simulink model "ChristophBessler"  (R2017a)
settings: Solver=VariableStepAuto  StartTime=0.0  StopTime=3  RelTol=1e-3
libraries: m3dof_library x12, dspindex x6
settings Model: Creator=Chris  LastModifiedBy=Chris

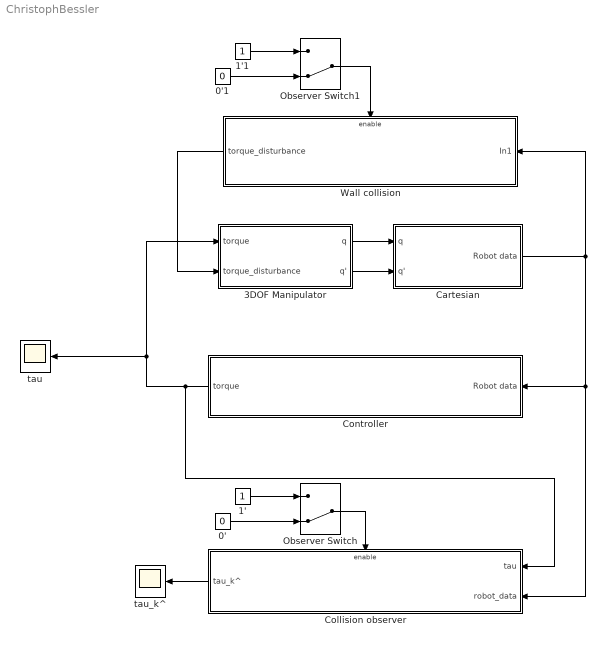
== system ChristophBessler ==
  0' : Constant  Value=0
  0'1 : Constant  Value=0
  1' : Constant
  1'1 : Constant
  3DOF Manipulator : Subsystem
  Cartesian : Subsystem
  Collision observer : Subsystem
  Controller : Subsystem
  Observer Switch : ManualSwitch  CurrentSetting=0
  Observer Switch1 : ManualSwitch  CurrentSetting=0
  Wall collision : Subsystem
  tau : Scope
  tau_k^ : Scope
  wires:
  3DOF Manipulator/1(q) -> Cartesian/1(q)
  3DOF Manipulator/2(q') -> Cartesian/2(q')
  Controller/1(torque) -> Collision observer/1(tau), tau/1, 3DOF Manipulator/1(torque)
  Collision observer/1(tau_k^) -> tau_k^/1
  Cartesian/1(Robot data) -> Wall collision/1(In1), Collision observer/2(robot_data), Controller/1(Robot data)
  Wall collision/1(torque_disturbance) -> 3DOF Manipulator/2(torque_disturbance)
  0'/1 -> Observer Switch/2
  1'/1 -> Observer Switch/1
  Observer Switch/1 -> Collision observer/Enable
  0'1/1 -> Observer Switch1/2
  Observer Switch1/1 -> Wall collision/Enable
  1'1/1 -> Observer Switch1/1

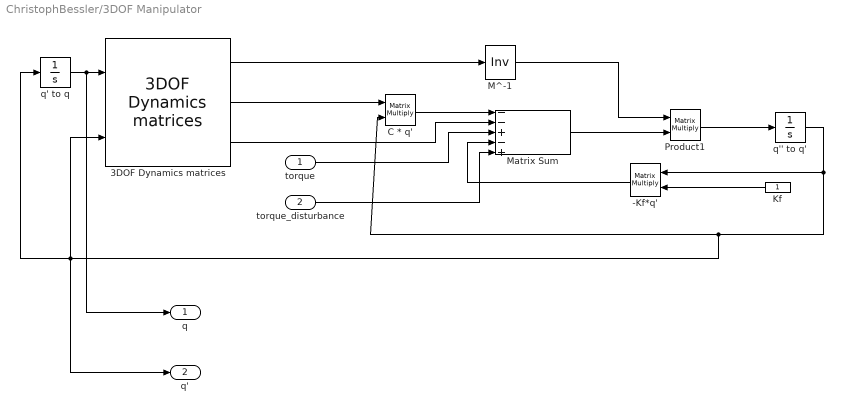
== system ChristophBessler/3DOF Manipulator ==
  torque : Inport
  torque_disturbance : Inport  Port=2
  -Kf*q' : Product  Multiplication=Matrix(*)
  3DOF Dynamics matrices : m3dof_library/3DOF Dynamics matrices  m1=m1  mX1=mx1  ZZ1=I1  m2=m2  mX2=mx2  ZZ2=I2  m3=m3  mX3=mx3  ZZ3=I3  a1=l1  a2=l2  a3=l3  eg=eg
  C * q' : Product  Multiplication=Matrix(*)
  Kf : Constant
  M^-1 : Product  Inputs=/  Multiplication=Matrix(*)
  Matrix Sum : Sum  Inputs=--+-+
  Product1 : Product  Multiplication=Matrix(*)
  q' to q : Integrator  InitialCondition=[3.66519; -0.523599; 0.349066]
  q'' to q' : Integrator
  q : Outport
  q' : Outport  Port=2
  wires:
  q' to q/1 -> q/1, 3DOF Dynamics matrices/1
  M^-1/1 -> Product1/1
  q'' to q'/1 -> -Kf*q'/1, C * q'/2, q'/1, q' to q/1, 3DOF Dynamics matrices/2
  3DOF Dynamics matrices/2 -> C * q'/1
  3DOF Dynamics matrices/1 -> M^-1/1
  Matrix Sum/1 -> Product1/2
  C * q'/1 -> Matrix Sum/1
  Product1/1 -> q'' to q'/1
  3DOF Dynamics matrices/3 -> Matrix Sum/2
  torque/1 -> Matrix Sum/3
  Kf/1 -> -Kf*q'/2
  -Kf*q'/1 -> Matrix Sum/4
  torque_disturbance/1 -> Matrix Sum/5

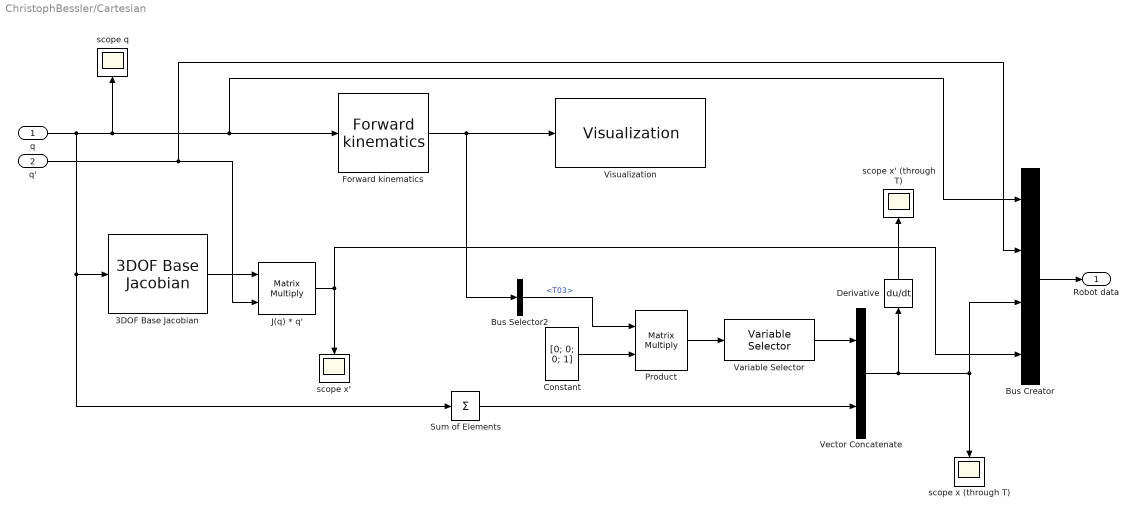
== system ChristophBessler/Cartesian ==
  q : Inport
  q' : Inport  Port=2
  3DOF Base Jacobian : m3dof_library/3DOF Base Jacobian  a1=l1  a2=l2  a3=l3
  Bus Creator : BusCreator  Inputs=4
  Bus Selector2 : BusSelector  OutputSignals=T03
  Constant : Constant  Value=[0; 0; 0; 1]  VectorParams1D=off
  Derivative : Derivative
  Forward kinematics : m3dof_library/Forward kinematics  a1=l1  a2=l2  a3=l3  alpha=0
  J(q) * q' : Product  Multiplication=Matrix(*)
  Product : Product  Multiplication=Matrix(*)
  Sum of Elements : Sum  Inputs=+
  Variable Selector : dspindex/Variable Selector  NumInputs=1  rowsOrCols=Rows  IdxMode=Fixed  Elements=[1 2]  ZerOneIdxMode=One-based  errmode=Clip Index  FillMode=off  FillValues=0
  Vector Concatenate : Concatenate
  Visualization : m3dof_library/Visualization  Ts0=1/16  al=1  a1=l1  a2=l2  a3=l3  alpha=0  eg=eg  tl=50
  scope q : Scope
  scope x (through T) : Scope
  scope x' : Scope
  scope x' (through T) : Scope
  Robot data : Outport
  wires:
  J(q) * q'/1 -> Bus Creator/4, scope x'/1
  3DOF Base Jacobian/1 -> J(q) * q'/1
  Forward kinematics/1 -> Bus Selector2/1, Visualization/1
  Constant/1 -> Product/2
  Variable Selector/1 -> Vector Concatenate/1
  Bus Selector2/1 -> Product/1  "<T03>"
  q/1 -> Sum of Elements/1, 3DOF Base Jacobian/1, Bus Creator/1, Forward kinematics/1, scope q/1
  q'/1 -> Bus Creator/2, J(q) * q'/2
  Vector Concatenate/1 -> Derivative/1, Bus Creator/3, scope x (through T)/1
  Derivative/1 -> scope x' (through T)/1
  Product/1 -> Variable Selector/1
  Bus Creator/1 -> Robot data/1
  Sum of Elements/1 -> Vector Concatenate/2

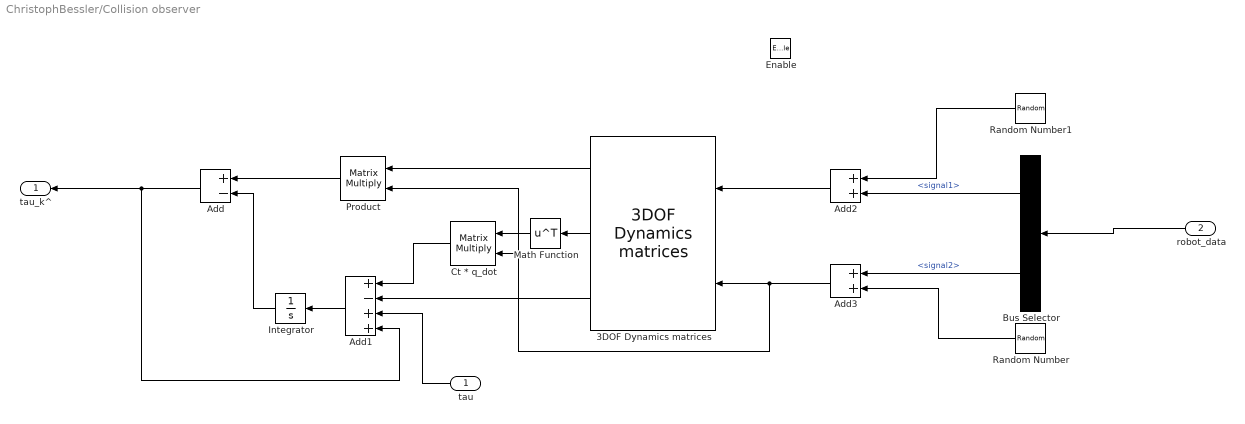
== system ChristophBessler/Collision observer ==
  tau : Inport
  robot_data : Inport  Port=2
  Enable : EnablePort
  3DOF Dynamics matrices : m3dof_library/3DOF Dynamics matrices  m1=m1  mX1=mx1  ZZ1=I1  m2=m2  mX2=mx2  ZZ2=I2  m3=m3  mX3=mx3  ZZ3=I3  a1=l1  a2=l2  a3=l3  eg=eg
  Add : Sum  Inputs=+-
  Add1 : Sum  Inputs=+-++
  Add2 : Sum
  Add3 : Sum
  Bus Selector : BusSelector  OutputSignals=signal1,signal2
  Ct * q_dot : Product  Multiplication=Matrix(*)
  Integrator : Integrator
  Math Function : Math  Operator=transpose  SaturateOnIntegerOverflow=on
  Product : Product  Multiplication=Matrix(*)
  Random Number : RandomNumber  Mean=1  Variance=0.001  SampleTime=0.1
  Random Number1 : RandomNumber  Variance=0.001  SampleTime=0.1
  tau_k^ : Outport
  wires:
  Add2/1 -> 3DOF Dynamics matrices/1
  Add3/1 -> Ct * q_dot/2, Product/2, 3DOF Dynamics matrices/2
  robot_data/1 -> Bus Selector/1
  3DOF Dynamics matrices/1 -> Product/1
  Product/1 -> Add/1
  3DOF Dynamics matrices/3 -> Add1/2
  tau/1 -> Add1/3
  Add1/1 -> Integrator/1
  Integrator/1 -> Add/2
  Bus Selector/1 -> Add2/2  "<signal1>"
  Bus Selector/2 -> Add3/1  "<signal2>"
  Random Number/1 -> Add3/2
  Random Number1/1 -> Add2/1
  3DOF Dynamics matrices/2 -> Math Function/1
  Math Function/1 -> Ct * q_dot/1
  Ct * q_dot/1 -> Add1/1
  Add/1 -> Add1/4, tau_k^/1

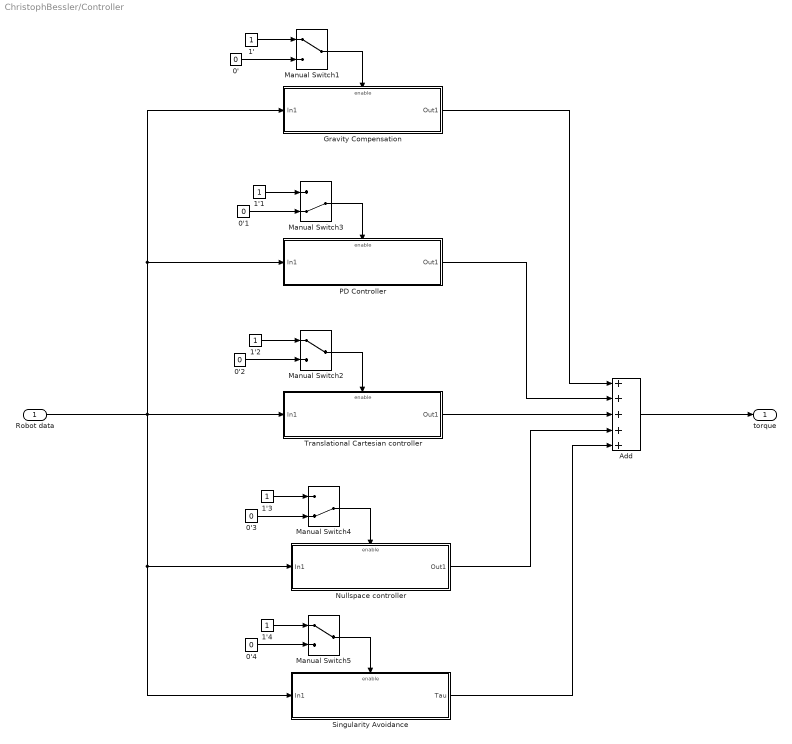
== system ChristophBessler/Controller ==
  Robot data : Inport
  0'{,1..4} (5 alike) : Constant  Value=0
  1'{,1..4} (5 alike) : Constant
  Add : Sum  Inputs=+++++
  Gravity Compensation : Subsystem
  Manual Switch1 : ManualSwitch
  Manual Switch2 : ManualSwitch
  Manual Switch3 : ManualSwitch  CurrentSetting=0
  Manual Switch4 : ManualSwitch  CurrentSetting=0
  Manual Switch5 : ManualSwitch
  Nullspace controller : Subsystem
  PD Controller : Subsystem
  Singularity Avoidance : Subsystem
  Translational Cartesian controller : Subsystem
  torque : Outport
  wires:
  Manual Switch1/1 -> Gravity Compensation/Enable
  Manual Switch3/1 -> PD Controller/Enable
  0'/1 -> Manual Switch1/2
  1'/1 -> Manual Switch1/1
  Add/1 -> torque/1
  1'1/1 -> Manual Switch3/1
  0'1/1 -> Manual Switch3/2
  Gravity Compensation/1(Out1) -> Add/1
  PD Controller/1(Out1) -> Add/2
  1'2/1 -> Manual Switch2/1
  0'2/1 -> Manual Switch2/2
  Manual Switch2/1 -> Translational Cartesian controller/Enable
  Translational Cartesian controller/1(Out1) -> Add/3
  Nullspace controller/1(Out1) -> Add/4
  0'3/1 -> Manual Switch4/2
  1'3/1 -> Manual Switch4/1
  1'4/1 -> Manual Switch5/1
  0'4/1 -> Manual Switch5/2
  Manual Switch4/1 -> Nullspace controller/Enable
  Manual Switch5/1 -> Singularity Avoidance/Enable
  Singularity Avoidance/1(Tau) -> Add/5
  Robot data/1 -> PD Controller/1(In1), Gravity Compensation/1(In1), Singularity Avoidance/1(In1), Nullspace controller/1(In1), Translational Cartesian controller/1(In1)

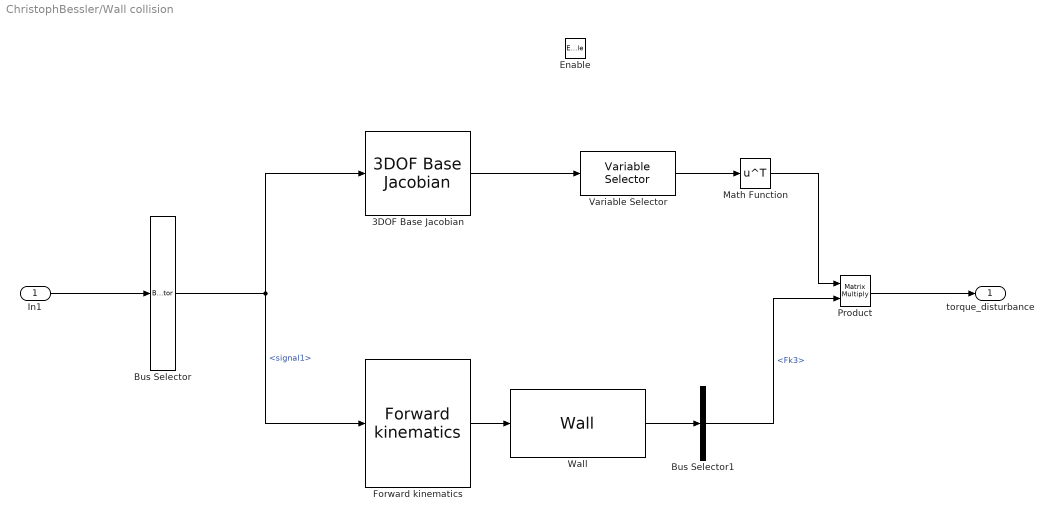
== system ChristophBessler/Wall collision ==
  In1 : Inport
  Enable : EnablePort
  3DOF Base Jacobian : m3dof_library/3DOF Base Jacobian  a1=l1  a2=l2  a3=l3
  Bus Selector : BusSelector  OutputSignals=signal1
  Bus Selector1 : BusSelector  OutputSignals=Fk3
  Forward kinematics : m3dof_library/Forward kinematics  a1=l1  a2=l2  a3=l3  alpha=0
  Math Function : Math  Operator=transpose  SaturateOnIntegerOverflow=on
  Product : Product  Multiplication=Matrix(*)
  Variable Selector : dspindex/Variable Selector  NumInputs=1  rowsOrCols=Rows  IdxMode=Fixed  Elements=[1 2]  ZerOneIdxMode=One-based  errmode=Clip Index  FillMode=on  FillValues=0
  Wall : m3dof_library/Wall  x0=[0 0]  w=[0 -1]
  torque_disturbance : Outport
  wires:
  In1/1 -> Bus Selector/1
  Bus Selector/1 -> Forward kinematics/1, 3DOF Base Jacobian/1  "<signal1>"
  Forward kinematics/1 -> Wall/1
  3DOF Base Jacobian/1 -> Variable Selector/1
  Variable Selector/1 -> Math Function/1
  Product/1 -> torque_disturbance/1
  Math Function/1 -> Product/1
  Wall/1 -> Bus Selector1/1
  Bus Selector1/1 -> Product/2  "<Fk3>"

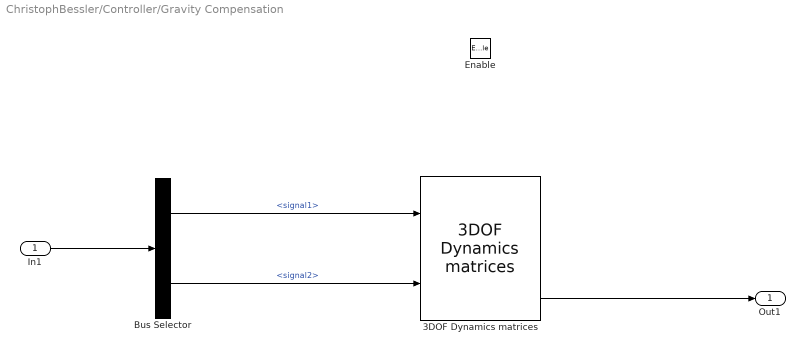
== system ChristophBessler/Controller/Gravity Compensation ==
  In1 : Inport
  Enable : EnablePort
  3DOF Dynamics matrices : m3dof_library/3DOF Dynamics matrices  m1=m1  mX1=mx1  ZZ1=I1  m2=m2  mX2=mx2  ZZ2=I2  m3=m3  mX3=mx3  ZZ3=I3  a1=l1  a2=l2  a3=l3  eg=eg
  Bus Selector : BusSelector  OutputSignals=signal1,signal2
  Out1 : Outport
  wires:
  In1/1 -> Bus Selector/1
  Bus Selector/2 -> 3DOF Dynamics matrices/2  "<signal2>"
  Bus Selector/1 -> 3DOF Dynamics matrices/1  "<signal1>"
  3DOF Dynamics matrices/3 -> Out1/1

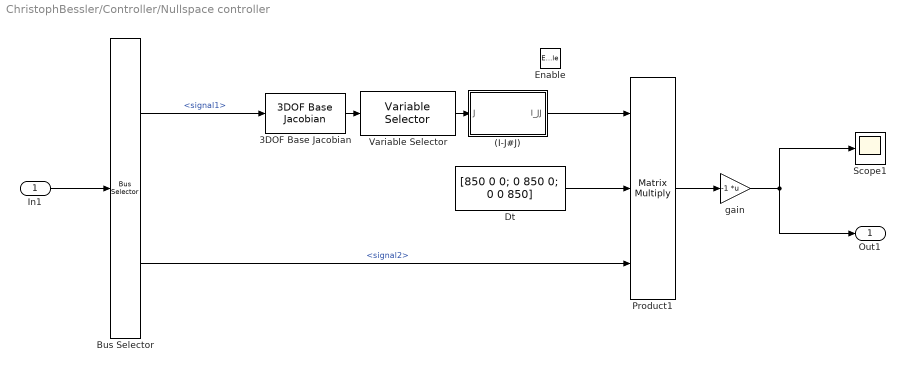
== system ChristophBessler/Controller/Nullspace controller ==
  In1 : Inport
  Enable : EnablePort
  (I-J#J) : MATLAB Function  TreatAsAtomicUnit=on
  3DOF Base Jacobian : m3dof_library/3DOF Base Jacobian  a1=l1  a2=l2  a3=l3
  Bus Selector : BusSelector  OutputSignals=signal1,signal2
  Dt : Constant  Value=[850 0 0; 0 850 0; 0 0 850]
  Product1 : Product  Inputs=3  Multiplication=Matrix(*)
  Scope1 : Scope
  Variable Selector : dspindex/Variable Selector  NumInputs=1  rowsOrCols=Rows  IdxMode=Fixed  Elements=[1 2]  ZerOneIdxMode=One-based  errmode=Clip Index  FillMode=on  FillValues=0
  "gain " : Gain  Gain=-1  Multiplication=Matrix(K*u)
  Out1 : Outport
  wires:
  In1/1 -> Bus Selector/1
  Product1/1 -> "gain "/1
  (I-J#J)/1(I_JJ) -> Product1/1
  "gain "/1 -> Scope1/1, Out1/1
  Bus Selector/1 -> 3DOF Base Jacobian/1  "<signal1>"
  Bus Selector/2 -> Product1/3  "<signal2>"
  Dt/1 -> Product1/2
  3DOF Base Jacobian/1 -> Variable Selector/1
  Variable Selector/1 -> (I-J#J)/1(J)

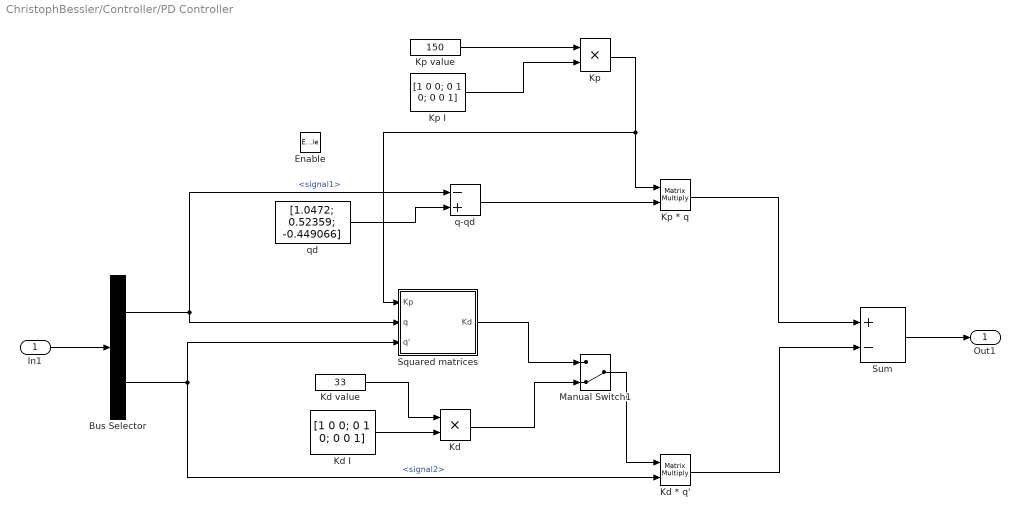
== system ChristophBessler/Controller/PD Controller ==
  In1 : Inport
  Enable : EnablePort
  Bus Selector : BusSelector  OutputSignals=signal1,signal2
  Kd : Product
  Kd * q' : Product  Multiplication=Matrix(*)
  Kd I : Constant  Value=[1 0 0; 0 1 0; 0 0 1]  VectorParams1D=off
  Kd value : Constant  Value=33
  Kp : Product
  Kp * q : Product  Multiplication=Matrix(*)
  Kp I : Constant  Value=[1 0 0; 0 1 0; 0 0 1]  VectorParams1D=off
  Kp value : Constant  Value=150
  Manual Switch1 : ManualSwitch  CurrentSetting=0
  Squared matrices : Subsystem
  Sum : Sum  Inputs=+-
  q-qd : Sum  Inputs=-+
  qd : Constant  Value=[1.0472; 0.52359; -0.449066]  VectorParams1D=off
  Out1 : Outport
  wires:
  In1/1 -> Bus Selector/1
  Bus Selector/1 -> Squared matrices/2(q), q-qd/1  "<signal1>"
  Bus Selector/2 -> Squared matrices/3(q'), Kd * q'/2  "<signal2>"
  Kp * q/1 -> Sum/1
  qd/1 -> q-qd/2
  q-qd/1 -> Kp * q/2
  Kd * q'/1 -> Sum/2
  Kp value/1 -> Kp/1
  Kd I/1 -> Kd/2
  Kd value/1 -> Kd/1
  Kp/1 -> Squared matrices/1(Kp), Kp * q/1
  Kp I/1 -> Kp/2
  Sum/1 -> Out1/1
  Kd/1 -> Manual Switch1/2
  Manual Switch1/1 -> Kd * q'/1
  Squared matrices/1(Kd) -> Manual Switch1/1

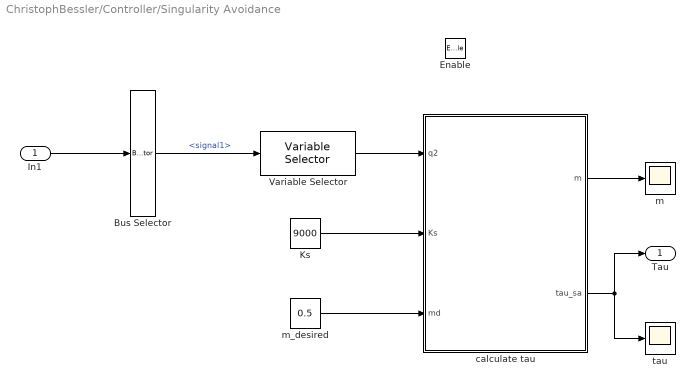
== system ChristophBessler/Controller/Singularity Avoidance ==
  In1 : Inport
  Enable : EnablePort
  Bus Selector : BusSelector  OutputSignals=signal1
  Ks : Constant  Value=9000
  Variable Selector : dspindex/Variable Selector  NumInputs=1  rowsOrCols=Rows  IdxMode=Fixed  Elements=[2]  ZerOneIdxMode=One-based  errmode=Clip Index  FillMode=on  FillValues=0
  calculate tau : MATLAB Function  TreatAsAtomicUnit=on
  m : Scope
  m_desired : Constant  Value=0.5
  tau : Scope
  Tau : Outport
  wires:
  In1/1 -> Bus Selector/1
  Ks/1 -> calculate tau/2(Ks)
  Variable Selector/1 -> calculate tau/1(q2)
  m_desired/1 -> calculate tau/3(md)
  calculate tau/2(tau_sa) -> tau/1, Tau/1
  Bus Selector/1 -> Variable Selector/1  "<signal1>"
  calculate tau/1(m) -> m/1

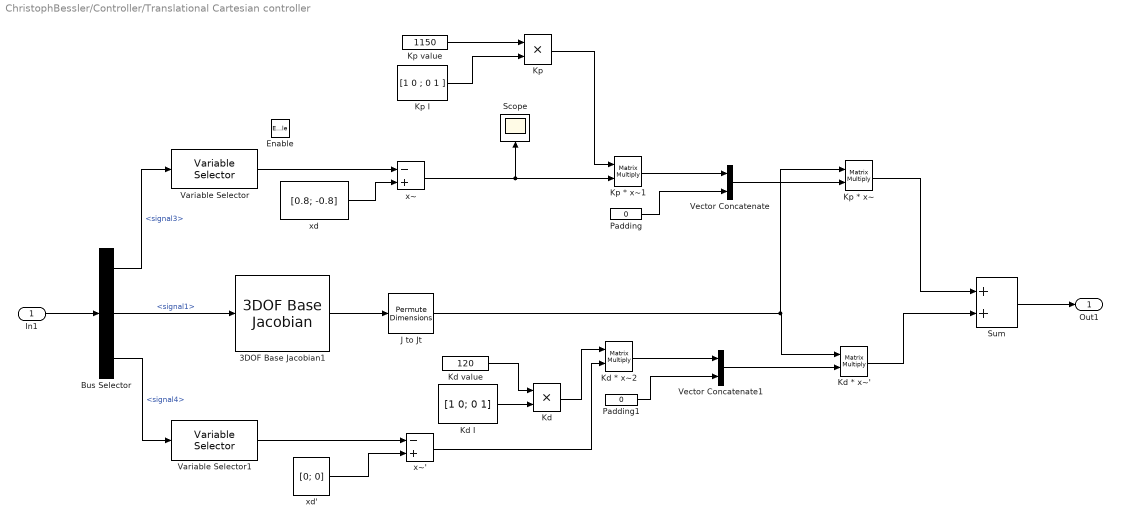
== system ChristophBessler/Controller/Translational Cartesian controller ==
  In1 : Inport
  Enable : EnablePort
  3DOF Base Jacobian1 : m3dof_library/3DOF Base Jacobian  a1=l1  a2=l2  a3=l3
  Bus Selector : BusSelector  OutputSignals=signal3,signal1,signal4
  J to Jt : PermuteDimensions
  Kd : Product
  Kd * x~' : Product  Multiplication=Matrix(*)
  Kd * x~2 : Product  Multiplication=Matrix(*)
  Kd I : Constant  Value=[1 0; 0 1]  VectorParams1D=off
  Kd value : Constant  Value=120
  Kp : Product
  Kp * x~ : Product  Multiplication=Matrix(*)
  Kp * x~1 : Product  Multiplication=Matrix(*)
  Kp I : Constant  Value=[1 0 ; 0 1 ]  VectorParams1D=off
  "Kp value " : Constant  Value=1150
  Padding : Constant  Value=0
  Padding1 : Constant  Value=0
  Scope : Scope
  Sum : Sum
  Variable Selector : dspindex/Variable Selector  NumInputs=1  rowsOrCols=Rows  IdxMode=Fixed  Elements=[1 2]  ZerOneIdxMode=One-based  errmode=Clip Index  FillMode=on  FillValues=0
  Variable Selector1 : dspindex/Variable Selector  NumInputs=1  rowsOrCols=Rows  IdxMode=Fixed  Elements=[1 2]  ZerOneIdxMode=One-based  errmode=Clip Index  FillMode=on  FillValues=0
  Vector Concatenate : Concatenate
  Vector Concatenate1 : Concatenate
  xd : Constant  Value=[0.8; -0.8]  VectorParams1D=off
  xd' : Constant  Value=[0; 0]  VectorParams1D=off
  x~ : Sum  Inputs=-+
  x~' : Sum  Inputs=-+
  Out1 : Outport
  wires:
  In1/1 -> Bus Selector/1
  xd/1 -> x~/2
  Kd * x~'/1 -> Sum/2
  Kd I/1 -> Kd/2
  Kd value/1 -> Kd/1
  Kp I/1 -> Kp/2
  Sum/1 -> Out1/1
  Bus Selector/2 -> 3DOF Base Jacobian1/1  "<signal1>"
  xd'/1 -> x~'/2
  3DOF Base Jacobian1/1 -> J to Jt/1
  Kp * x~/1 -> Sum/1
  J to Jt/1 -> Kp * x~/1, Kd * x~'/1
  Kp/1 -> Kp * x~1/1
  Variable Selector/1 -> x~/1
  Bus Selector/1 -> Variable Selector/1  "<signal3>"
  Variable Selector1/1 -> x~'/1
  Bus Selector/3 -> Variable Selector1/1  "<signal4>"
  Padding/1 -> Vector Concatenate/2
  x~/1 -> Scope/1, Kp * x~1/2
  Kp * x~1/1 -> Vector Concatenate/1
  Vector Concatenate/1 -> Kp * x~/2
  Padding1/1 -> Vector Concatenate1/2
  Vector Concatenate1/1 -> Kd * x~'/2
  Kd * x~2/1 -> Vector Concatenate1/1
  Kd/1 -> Kd * x~2/1
  x~'/1 -> Kd * x~2/2
  "Kp value "/1 -> Kp/1

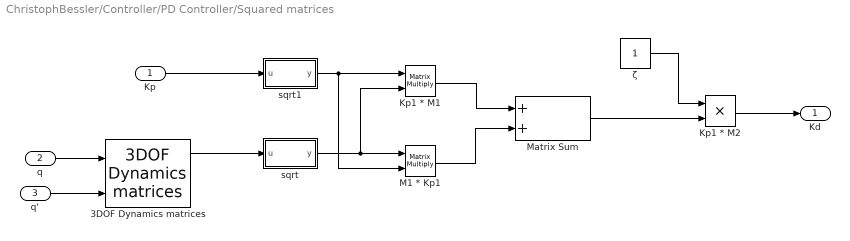
== system ChristophBessler/Controller/PD Controller/Squared matrices ==
  Kp : Inport
  q : Inport  Port=2
  q' : Inport  Port=3
  3DOF Dynamics matrices : m3dof_library/3DOF Dynamics matrices  m1=m1  mX1=mx1  ZZ1=I1  m2=m2  mX2=mx2  ZZ2=I2  m3=m3  mX3=mx3  ZZ3=I3  a1=l1  a2=l2  a3=l3  eg=eg
  Kp1 * M1 : Product  Multiplication=Matrix(*)
  Kp1 * M2 : Product
  M1 * Kp1 : Product  Multiplication=Matrix(*)
  Matrix Sum : Sum
  sqrt : MATLAB Function  TreatAsAtomicUnit=on
  sqrt1 : MATLAB Function  TreatAsAtomicUnit=on
  ζ : Constant
  Kd : Outport
  wires:
  q/1 -> 3DOF Dynamics matrices/1
  Kp/1 -> sqrt1/1(u)
  q'/1 -> 3DOF Dynamics matrices/2
  3DOF Dynamics matrices/1 -> sqrt/1(u)
  sqrt1/1(y) -> M1 * Kp1/2, Kp1 * M1/1
  sqrt/1(y) -> M1 * Kp1/1, Kp1 * M1/2
  Kp1 * M1/1 -> Matrix Sum/1
  M1 * Kp1/1 -> Matrix Sum/2
  Kp1 * M2/1 -> Kd/1
  Matrix Sum/1 -> Kp1 * M2/2
  ζ/1 -> Kp1 * M2/1

== matlab function ChristophBessler/Controller/PD Controller/Squared matrices/sqrt1 ==
  data: u input; y output
function y = fcn(u)

y = real(sqrt(u));

== matlab function ChristophBessler/Controller/PD Controller/Squared matrices/sqrt ==
  data: u input; y output
function y = fcn(u)

y = real(sqrt(u));

== matlab function ChristophBessler/Controller/Nullspace controller/(I-J#J) ==
  data: J input; I_JJ output
function I_JJ = fcn(J)

I_JJ = eye(3)-J'*pinv(J)';

== matlab function ChristophBessler/Controller/Singularity Avoidance/calculate tau ==
  data: q2 input; m output; Ks input; md input; tau_sa output
function [m,tau_sa] = singularity_avoidance(q2,Ks,md)

% Constants
l1 = 1/3;
l2 = 1/3;
L = l1*l2;

% calculate m
m = abs(sin(q2)*L);

% calculate torque for singularity avoidance
if m < md %smaller than desired manipulability
    tau_sa2 = Ks*(md-m)*cos(q2)*sign(sin(q2))*L;
else
    tau_sa2 = 0;
end

tau_sa = [0; tau_sa2; 0];
